simulink model "msfcndemo_varpulse"  (Simulink 7.6)
settings: Solver=VariableStepDiscrete  StartTime=0.0  StopTime=20  MaxStep=0.4  RelTol=1e-3
Description:
  | Creates a Variable Pulse Generator by using an S-function to control
  | the pulse width of a Pulse Generator block.
settings Model: Creator=The MathWorks Inc.
settings DataIOCC: SaveOutput=off  SignalLogging=off
settings OptimizationCC: InitFltsAndDblsToZero=on
settings DebuggingCC: SaveWithParameterizedLinksMsg=none  SignalResolutionControl=TryResolveAllWithWarning  MultiTaskDSMMsg=warning  MultiTaskCondExecSysMsg=none
settings SFSimCC: SimParseCustomCode=off
settings RTWCC: IncludeERTFirstTime=on
settings GRTTargetCC: TargetFcnLib=ansi_tfl_tmw.mat

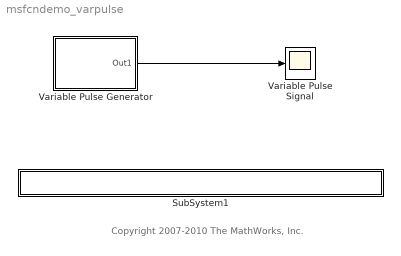
== system msfcndemo_varpulse ==
  note: Copyright 2007-2010 The MathWorks, Inc.
  SubSystem1 : Subsystem  mask{filename=msfcn_varpulse.m}
      mask init:
      | x=sfundemo_maskdisp;
      settings: AttributesFormatString=\n  OpenFcn=sfundemo_openfcn
      mask Display: disp(['MATLAB file: ' x]);
  Variable Pulse Signal : Scope
      settings: TimeRange=20  YMin=-1  YMax=2
  Variable Pulse Generator : Subsystem
      mask Display:
      | plot([0 .05 .05 .2 .2 .3 .3 .35 .35 .525 .525 .9 .9 1], ...
      | [0 0 1 1 0 0 1 1 0 0 1 1 0 0])
  wires:
  Variable Pulse Generator/1(Out1) -> Variable Pulse Signal/1

== system msfcndemo_varpulse/SubSystem1 ==

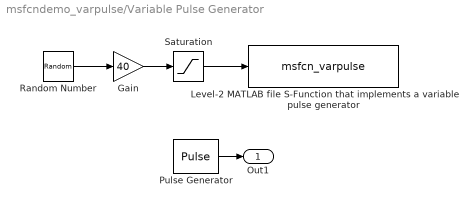
== system msfcndemo_varpulse/Variable Pulse Generator ==
  Gain : Gain  Gain=40
  Level-2 MATLAB file S-Function that implements a variable pulse generator : M-S-Function  FunctionName=msfcn_varpulse
  Pulse Generator : DiscretePulseGenerator  PulseType=Time based  PulseWidth=0.1
  Random Number : RandomNumber  SampleTime=0
  Saturation : Saturate  UpperLimit=100  LowerLimit=0.1
  Out1 : Outport
  wires:
  Random Number/1 -> Gain/1
  Gain/1 -> Saturation/1
  Saturation/1 -> Level-2 MATLAB file S-Function that implements a variable pulse generator/1
  Pulse Generator/1 -> Out1/1
